simulink model "ex_11_1"  (Simulink 6.3)
settings: Solver=ode45  StartTime=0.0  StopTime=2.0  RelTol=1e-3
settings Model: LastModifiedBy=Yuantao Gu

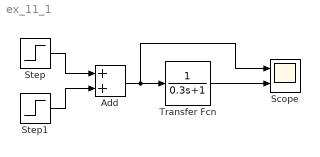
== system ex_11_1 ==
  Add : Sum  OutScaling=2^-10
  Scope : Scope  NumInputPorts=2
      settings: YMin=-5~-5  YMax=5~5
  Step : Step  StopFcn=disp('stoped!')  Time=0  SampleTime=0
  Step1 : Step  StopFcn=disp('stoped!')  Time=0.5  After=-1  SampleTime=0
  Transfer Fcn : TransferFcn  Denominator=[0.3 1]
  wires:
  Transfer Fcn/1 -> Scope/2
  Add/1 -> Transfer Fcn/1, Scope/1
  Step/1 -> Add/1
  Step1/1 -> Add/2
